simulink model "fec_ber_hw_V2"  (R2020b)
settings: Solver=FixedStepDiscrete  StartTime=0.0  StopTime=T  RelTol=1e-3
values from neighbouring files (symbols this model uses):
  aximm_awgn_reset = 0    [setup.m]
  aximm_bit_count_reset = 0    [setup.m]
  aximm_bits = n_blocks * k    (= 80)    [setup.m]
  aximm_ctrl_word_dec = 0    [setup.m]
  aximm_ctrl_word_enc = 0    [setup.m]
  aximm_enable = 1    [setup.m]
  aximm_length = k * n_blocks    (= 80)    [setup.m]
  aximm_length_dec = n    (= 160)    [setup.m]
  aximm_length_enc = k    (= 80)    [setup.m]
  aximm_llr_mag_reset = 0    [setup.m]
  aximm_llr_scale = (1/noise_var) * llr_scale    (= 1000)    [setup.m]
  aximm_load_dec = 1    [setup.m]
  aximm_load_enc = 1    [setup.m]
  aximm_noise_std = sqrt(noise_var)    [setup.m]
  aximm_reset = 0    [setup.m]
  d = sqrt(-2*log([0:1/4095:1]))    [setup.m]
  fs = 160e6    (= 160000000)    [setup.m]
  generator_polynomial = '''z^13 + z^12 + z^11 + z^8 + 1'''    [setup.m]
  llr_scale = 7.75/7.75    (= 1)    [setup.m]
libraries: simulink x931, hdlsllib x419, commseqgen3 x52, dspsigops x22, commblkcod2 x3, lib_rfsoc_fec x2
(part 1 of 47)
settings Model: Creator=ckb13136  LastModifiedBy=LDM
settings OptimizationCC: BlockReduction=off  ConditionallyExecuteInputs=off  DefaultParameterBehavior=Inlined
settings DebuggingCC: AlgebraicLoopMsg=error  SingleTaskRateTransMsg=error
settings HardwareCC: ProdBitPerPointer=32  ProdBitPerSizeT=32  ProdBitPerPtrDiffT=32  ProdLargestAtomicFloat=None  ProdIntDivRoundTo=Undefined  ProdEndianess=Unspecified  ProdWordSize=32  ProdHWDeviceType=ASIC/FPGA->ASIC/FPGA  TargetBitPerPointer=64  TargetBitPerSizeT=64  TargetBitPerPtrDiffT=64  TargetLongLongMode=on  TargetIntDivRoundTo=Zero  TargetEndianess=LittleEndian  TargetWordSize=64  TargetHWDeviceType=Custom Processor->MATLAB Host Computer  ProdEqTarget=off

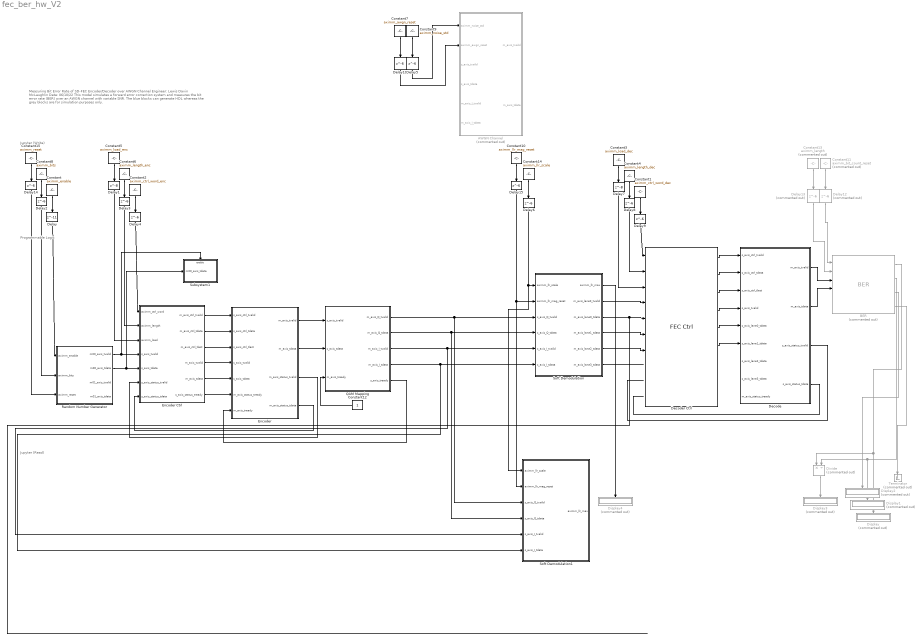
== system fec_ber_hw_V2 ==
  note: Measuring Bit Error Rate of SD-FEC Encoder/Decoder over AWGN Channel
      | Engineer: Lewis Davin McLaughlin
      | Date: 06/10/22
      |
      | This model simulates a forward error correction system and measures the bit error rate (BER) over an AWGN channel with variable SNR. The blue blocks can generate HDL whereas the grey blocks are for simulation purposes only.
  note: Jupyter (Write)
  note: Programmable Logic
  note: Jupyter (Read)
  AWGN Channel : Subsystem  Commented=on  AncestorBlock=lib_rfsoc_fec/AWGN Channel  TreatAsAtomicUnit=on
  BER : lib_rfsoc_fec/BER  Commented=on  SystemSampleTime=-1  VariantActivationTime=update diagram  Latency=0  AutoFrameSizeCalculation=off
  Constant : Constant  Value=aximm_enable  OutDataTypeStr=uint32  SampleTime=1/fs
  Constant1 : Constant  Value=aximm_ctrl_word_dec  OutDataTypeStr=uint32  SampleTime=1/fs
  Constant10 : Constant  Value=aximm_llr_mag_reset  OutDataTypeStr=uint32  SampleTime=1/(fs)
  Constant11 : Constant  Commented=on  Value=aximm_bit_count_reset  OutDataTypeStr=uint32  SampleTime=1/(fs*16)
  Constant12 : Constant  OutDataTypeStr=boolean  SampleTime=1/(fs)
  Constant13 : Constant  Commented=on  Value=aximm_length  OutDataTypeStr=uint32  SampleTime=1/(fs*16)
  Constant14 : Constant  Value=aximm_llr_scale  OutDataTypeStr=fixdt(0,32,22)  SampleTime=1/(fs)
  Constant15 : Constant  Value=aximm_reset  OutDataTypeStr=uint32  SampleTime=1/fs
  Constant2 : Constant  Value=aximm_ctrl_word_enc  OutDataTypeStr=uint32  SampleTime=1/fs
  Constant3 : Constant  Value=aximm_load_dec  OutDataTypeStr=uint32  SampleTime=1/fs
  Constant4 : Constant  Value=aximm_length_dec  OutDataTypeStr=uint32  SampleTime=1/fs
  Constant5 : Constant  Value=aximm_load_enc  OutDataTypeStr=uint32  SampleTime=1/fs
  Constant6 : Constant  Value=aximm_length_enc  OutDataTypeStr=uint32  SampleTime=1/fs
  Constant7 : Constant  Value=aximm_awgn_reset  OutDataTypeStr=uint32  SampleTime=1/(fs*2)
  Constant8 : Constant  Value=aximm_bits  OutDataTypeStr=uint32  SampleTime=1/fs
  Constant9 : Constant  Value=aximm_noise_std  OutDataTypeStr=fixdt(0,32,30)  SampleTime=1/(fs*2)
  Decode : Subsystem
  Decoder Ctrl : lib_rfsoc_fec/FEC Ctrl  SystemSampleTime=-1  VariantActivationTime=update diagram  Latency=0  AutoFrameSizeCalculation=off
  Delay : Delay  DelayLength=11
  Delay1 : Delay  DelayLength=8
  Delay{2..6,8..10,14..15} (10 alike) : Delay  DelayLength=6
  Delay12 : Delay  Commented=on  DelayLength=6
  Delay13 : Delay  Commented=on  DelayLength=6
  Delay7 : Delay  DelayLength=8
  Display{,1..4} (5 alike) : Display  Commented=on
  Divide : Product  Commented=on  Inputs=*/
  Encoder : Subsystem
  Encoder Ctrl : Subsystem  AncestorBlock=lib_rfsoc_fec/FEC Ctrl  TreatAsAtomicUnit=on
  QAM Mapping : Subsystem  AncestorBlock=lib_rfsoc_fec/QAM Mapping  TreatAsAtomicUnit=on
  Random Number Generator : Subsystem  AncestorBlock=lib_rfsoc_fec/Random Number Generator  TreatAsAtomicUnit=on
  Soft Demodulation : Subsystem  AncestorBlock=lib_rfsoc_fec/Soft Demodulation  TreatAsAtomicUnit=on
  Soft Demodulation1 : Subsystem  AncestorBlock=lib_rfsoc_fec/Soft Demodulation  TreatAsAtomicUnit=on
  Subsystem1 : Subsystem
  Terminator : Terminator  Commented=on
  wires:
  BER/3 -> Display2/1
  Soft Demodulation/1(aximm_llr_max) -> Display4/1
  Constant6/1 -> Delay3/1
  Constant7/1 -> Delay10/1
  Encoder Ctrl/2(m_axis_ctrl_tdata) -> Encoder/2(s_axis_ctrl_tdata)
  Constant12/1 -> QAM Mapping/3(m_axis_tready)
  Constant/1 -> Delay/1
  Delay15/1 -> Soft Demodulation1/2(aximm_llr_mag_reset), Soft Demodulation/2(aximm_llr_mag_reset)
  Constant10/1 -> Delay15/1
  Delay10/1 -> AWGN Channel/2(aximm_awgn_reset)
  Delay/1 -> Random Number Generator/1(aximm_enable)
  Delay3/1 -> Encoder Ctrl/2(aximm_length)
  Delay2/1 -> Random Number Generator/2(aximm_bits)
  BER/1 -> Divide/1, Display/1
  Soft Demodulation/2(m_axis_lane0_tvalid) -> Decoder Ctrl/4
  Delay12/1 -> BER/1
  Constant11/1 -> Delay12/1
  BER/2 -> Divide/2, Display1/1
  Encoder Ctrl/5(m_axis_tdata) -> Encoder/5(s_axis_tdata)
  Decoder Ctrl/4 -> Decode/4(s_axis_tvalid)
  Constant2/1 -> Delay4/1
  Constant9/1 -> Delay5/1
  Decode/1(m_axis_tvalid) -> BER/3
  Delay1/1 -> Encoder Ctrl/3(aximm_load)
  Delay4/1 -> Encoder Ctrl/1(aximm_ctrl_word)
  Decode/2(m_axis_tdata) -> BER/4
  Decoder Ctrl/2 -> Decode/2(s_axis_ctrl_tdata)
  Encoder Ctrl/3(m_axis_ctrl_tlast) -> Encoder/3(s_axis_ctrl_tlast)
  Decoder Ctrl/3 -> Decode/3(s_axis_ctrl_tlast)
  Divide/1 -> Display3/1
  Encoder/1(m_axis_tvalid) -> QAM Mapping/1(s_axis_tvalid)
  Delay6/1 -> Soft Demodulation1/1(aximm_llr_scale), Soft Demodulation/1(aximm_llr_scale)
  Encoder Ctrl/4(m_axis_tvalid) -> Encoder/4(s_axis_tvalid)
  Delay5/1 -> AWGN Channel/1(aximm_noise_std)
  Encoder/2(m_axis_tdata) -> QAM Mapping/2(s_axis_tdata)
  Decoder Ctrl/1 -> Decode/1(s_axis_ctrl_tvalid)
  Constant14/1 -> Delay6/1
  Decoder Ctrl/5 -> Decode/5(s_axis_lane0_tdata)
  Constant8/1 -> Delay2/1
  Encoder Ctrl/1(m_axis_ctrl_tvalid) -> Encoder/1(s_axis_ctrl_tvalid)
  Constant5/1 -> Delay1/1
  BER/4 -> Terminator/1
  Constant13/1 -> Delay13/1
  Delay13/1 -> BER/2
  Delay14/1 -> Random Number Generator/3(aximm_reset)
  Constant15/1 -> Delay14/1
  QAM Mapping/5(s_axis_tready) -> Encoder/7(m_axis_tready)
  Random Number Generator/2(m00_axis_tdata) -> Subsystem1/1(m00_axis_tdata), Encoder Ctrl/5(s_axis_tdata)
  Random Number Generator/1(m00_axis_tvalid) -> Subsystem1/Enable, Encoder Ctrl/4(s_axis_tvalid)
  Encoder Ctrl/6(s_axis_status_tready) -> Encoder/6(m_axis_status_tready)
  QAM Mapping/1(m_axis_Q_tvalid) -> Soft Demodulation1/3(s_axis_Q_tvalid), Soft Demodulation/3(s_axis_Q_tvalid)
  QAM Mapping/2(m_axis_Q_tdata) -> Soft Demodulation1/4(s_axis_Q_tdata), Soft Demodulation/4(s_axis_Q_tdata)
  QAM Mapping/3(m_axis_I_tvalid) -> Soft Demodulation1/5(s_axis_I_tvalid), Soft Demodulation/5(s_axis_I_tvalid)
  QAM Mapping/4(m_axis_I_tdata) -> Soft Demodulation1/6(s_axis_I_tdata), Soft Demodulation/6(s_axis_I_tdata)
  Encoder/3(m_axis_status_tvalid) -> Encoder Ctrl/6(s_axis_status_tvalid)
  Encoder/4(m_axis_status_tdata) -> Encoder Ctrl/7(s_axis_status_tdata)
  Soft Demodulation/4(m_axis_lane1_tdata) -> Decoder Ctrl/6
  Soft Demodulation/5(m_axis_lane2_tdata) -> Decoder Ctrl/7
  Soft Demodulation/6(m_axis_lane3_tdata) -> ?
  Delay9/1 -> Decoder Ctrl/1
  Constant4/1 -> Delay8/1
  Constant1/1 -> Delay9/1
  Constant3/1 -> Delay7/1
  Delay8/1 -> Decoder Ctrl/2
  Delay7/1 -> Decoder Ctrl/3
  Decoder Ctrl/6 -> Decode/6(s_axis_lane1_tdata)
  ? -> Decode/7(s_axis_lane2_tdata)
  ? -> Decode/8(s_axis_lane3_tdata)
  Decode/3(s_axis_status_tvalid) -> ?
  Decode/4(s_axis_status_tdata) -> ?
  Soft Demodulation/3(m_axis_lane0_tdata) -> Decoder Ctrl/5

== system fec_ber_hw_V2/AWGN Channel ==
  aximm_noise_std : Inport
  aximm_awgn_reset : Inport  Port=2
  s_axis_tvalid : Inport  Port=3
  s_axis_tdata : Inport  Port=4
  m_axis_I_tvalid : Inport  Port=5
  m_axis_I_tdata : Inport  Port=6
  AWGN Generator : Subsystem
  Add : Sum  OutDataTypeStr=fixdt(1,16,11)  SaturateOnIntegerOverflow=on
  Bit Concat : hdlsllib/Logic and Bit Operations/Bit Concat  numInputs=2
  Bit Slice : hdlsllib/Logic and Bit Operations/Bit Slice  lidx=3  ridx=0
      settings: SourceProductBaseCode=SL
  Bit Slice1 : hdlsllib/Logic and Bit Operations/Bit Slice  lidx=7  ridx=4
      settings: SourceProductBaseCode=SL
  Cast To Boolean : DataTypeConversion  OutDataTypeStr=boolean
  Complex to Real-Imag : ComplexToRealImag
  Data Type Conversion : DataTypeConversion  OutDataTypeStr=fixdt(1,4,0)  ConvertRealWorld=Stored Integer (SI)
  Data Type Conversion1 : DataTypeConversion  OutDataTypeStr=fixdt(1,4,0)  ConvertRealWorld=Stored Integer (SI)
  Delay{,1..5} (6 alike) : Delay
  Downsample{,1..3} (4 alike) : DownSample  N=4  RateOptions=Allow multirate processing
  Real-Imag to Complex : RealImagToComplex
  Repeat : dspsigops/Repeat  N=4  InputProcessing=Columns as channels (frame based)  RateOptions=Allow multirate processing  ic=0  mode=Unused parameter value
      settings: SourceProductName=DSP System Toolbox
  Repeat1 : dspsigops/Repeat  N=4  InputProcessing=Columns as channels (frame based)  RateOptions=Allow multirate processing  ic=0  mode=Unused parameter value
      settings: SourceProductName=DSP System Toolbox
  sample_and_hold : Subsystem
  m_axis_tvalid : Outport
  m_axis_tdata : Outport  Port=2
  wires:
  Cast To Boolean/1 -> Downsample3/1
  aximm_awgn_reset/1 -> Cast To Boolean/1
  Downsample3/1 -> Delay5/1
  Complex to Real-Imag/2 -> Bit Concat/2
  Complex to Real-Imag/1 -> Bit Concat/1
  Bit Concat/1 -> Delay4/1
  Add/1 -> Complex to Real-Imag/1
  Real-Imag to Complex/1 -> Add/1
  Data Type Conversion1/1 -> Real-Imag to Complex/2
  Data Type Conversion/1 -> Real-Imag to Complex/1
  Bit Slice/1 -> Data Type Conversion1/1
  Bit Slice1/1 -> Data Type Conversion/1
  Delay4/1 -> Repeat1/1
  Delay3/1 -> Repeat/1
  Repeat/1 -> m_axis_tvalid/1
  Repeat1/1 -> m_axis_tdata/1
  Delay1/1 -> Bit Slice/1, Bit Slice1/1
  s_axis_tdata/1 -> sample_and_hold/2(data_in)
  s_axis_tvalid/1 -> sample_and_hold/1(valid_in)
  sample_and_hold/2(" data_out") -> Downsample/1
  Delay/1 -> Delay3/1
  Downsample/1 -> Delay1/1
  Downsample1/1 -> Delay/1
  sample_and_hold/1(" valid_out") -> Downsample1/1
  Delay5/1 -> AWGN Generator/2(reset)
  Downsample2/1 -> Delay2/1
  Delay2/1 -> AWGN Generator/1(noise_std)
  aximm_noise_std/1 -> Downsample2/1
  AWGN Generator/1(awgn) -> Add/2

== system fec_ber_hw_V2/Decode ==
  s_axis_ctrl_tvalid : Inport
  s_axis_ctrl_tdata : Inport  Port=2
  s_axis_ctrl_tlast : Inport  Port=3
  s_axis_tvalid : Inport  Port=4
  s_axis_lane0_tdata : Inport  Port=5
  s_axis_lane1_tdata : Inport  Port=6
  s_axis_lane2_tdata : Inport  Port=7
  s_axis_lane3_tdata : Inport  Port=8
  m_axis_status_tready : Inport  Port=9
  Bit Slice{,2,4,6} (4 alike) : hdlsllib/Logic and Bit Operations/Bit Slice  lidx=63  ridx=0
      settings: SourceProductBaseCode=SL
  Bit Slice{1,3,5,7} (4 alike) : hdlsllib/Logic and Bit Operations/Bit Slice  lidx=127  ridx=64
      settings: SourceProductBaseCode=SL
  Cast To Boolean : DataTypeConversion  OutDataTypeStr=boolean
  Constant1 : Constant  Value=aximm_bits  OutDataTypeStr=uint32  SampleTime=1/fs
  Constant3 : Constant  Value=0  OutDataTypeStr=uint32  SampleTime=1/(16*fs)
  Constant4 : Constant  Value=0  OutDataTypeStr=boolean  SampleTime=1/(16*fs)
  Constant8 : Constant  Value=aximm_bits  OutDataTypeStr=uint32  SampleTime=1/fs
  Data Type Conversion : DataTypeConversion  OutDataTypeStr=fixdt(1,6,2)  ConvertRealWorld=Stored Integer (SI)
  Gain : Gain  Gain=1/llr_scale
  MATLAB Function3 : MATLAB Function  TreatAsAtomicUnit=on
  MATLAB Function5 : MATLAB Function  TreatAsAtomicUnit=on
  NOT2 : Logic  Operator=NOT  IconShape=distinctive  AllPortsSameDT=off  OutDataTypeStr=boolean
  Subsystem : Subsystem
  Subsystem1 : Subsystem
  Terminator{,1..3} (4 alike) : Terminator
  m_axis_tvalid : Outport
  m_axis_tdata : Outport  Port=2
  s_axis_status_tvalid : Outport  Port=3
  s_axis_status_tdata : Outport  Port=4
  wires:
  Data Type Conversion/1 -> Gain/1
  ? -> Data Type Conversion/1
  Gain/1 -> ?
  s_axis_ctrl_tvalid/1 -> Terminator/1
  s_axis_ctrl_tdata/1 -> Terminator1/1
  s_axis_ctrl_tlast/1 -> Terminator2/1
  m_axis_status_tready/1 -> Terminator3/1
  Constant4/1 -> s_axis_status_tvalid/1
  Constant3/1 -> s_axis_status_tdata/1
  NOT2/1 -> MATLAB Function5/3(frame)
  Subsystem/1(Out1) -> NOT2/1
  s_axis_tvalid/1 -> MATLAB Function3/2(valid)
  Constant8/1 -> MATLAB Function3/1(bits)
  MATLAB Function3/2(frame_out) -> Subsystem/1(In1)
  MATLAB Function3/1(valid_out) -> Cast To Boolean/1
  Bit Slice/1 -> MATLAB Function3/3(lane_0)
  Bit Slice1/1 -> MATLAB Function3/4(lane_1)
  s_axis_lane0_tdata/1 -> Bit Slice1/1, Bit Slice/1
  s_axis_lane1_tdata/1 -> Bit Slice2/1, Bit Slice3/1
  Bit Slice3/1 -> MATLAB Function3/6(lane_3)
  Bit Slice2/1 -> MATLAB Function3/5(lane_2)
  s_axis_lane2_tdata/1 -> Bit Slice5/1, Bit Slice4/1
  Bit Slice4/1 -> MATLAB Function3/7(lane_4)
  Bit Slice5/1 -> MATLAB Function3/8(lane_5)
  Bit Slice7/1 -> MATLAB Function3/10(lane_7)
  Bit Slice6/1 -> MATLAB Function3/9(lane_6)
  s_axis_lane3_tdata/1 -> Bit Slice7/1, Bit Slice6/1
  Constant1/1 -> MATLAB Function5/1(bits)
  MATLAB Function5/1(tvalid) -> Subsystem1/Enable
  MATLAB Function5/2(lane_0) -> Subsystem1/1(lane_0)
  Cast To Boolean/1 -> MATLAB Function5/2(valid), Subsystem/Enable

== system fec_ber_hw_V2/Encoder ==
  s_axis_ctrl_tvalid : Inport
  s_axis_ctrl_tdata : Inport  Port=2
  s_axis_ctrl_tlast : Inport  Port=3
  s_axis_tvalid : Inport  Port=4
  s_axis_tdata : Inport  Port=5
  m_axis_status_tready : Inport  Port=6
  m_axis_tready : Inport  Port=7
  Cast To Double : DataTypeConversion  OutDataTypeStr=double
  Constant1 : Constant  Value=aximm_bits * 2  OutDataTypeStr=uint32  SampleTime=1/(fs)
  Constant2 : Constant  Value=0  OutDataTypeStr=boolean  SampleTime=1/fs
  Constant3 : Constant  Commented=on  Value=aximm_bits  OutDataTypeStr=uint32  SampleTime=1/fs
  Constant4 : Constant  Value=0  OutDataTypeStr=boolean  SampleTime=1/fs
  Constant8 : Constant  Value=aximm_bits  OutDataTypeStr=uint32  SampleTime=1/(fs)
  Encode : Subsystem
  MATLAB Function : MATLAB Function  Commented=on  TreatAsAtomicUnit=on
  MATLAB Function3 : MATLAB Function  TreatAsAtomicUnit=on
  MATLAB Function4 : MATLAB Function  TreatAsAtomicUnit=on
  MATLAB Function5 : MATLAB Function  Commented=on  TreatAsAtomicUnit=on
  NOT2 : Logic  Commented=on  Operator=NOT  IconShape=distinctive  AllPortsSameDT=off  OutDataTypeStr=boolean
  Subsystem : Subsystem  Commented=on
  Subsystem1 : Subsystem  Commented=on
  Terminator{,1..4} (5 alike) : Terminator
  m_axis_tvalid : Outport
  m_axis_tdata : Outport  Port=2
  m_axis_status_tvalid : Outport  Port=3
  m_axis_status_tdata : Outport  Port=4
  wires:
  Constant4/1 -> m_axis_status_tvalid/1
  s_axis_ctrl_tvalid/1 -> Terminator/1
  s_axis_ctrl_tdata/1 -> Terminator1/1
  s_axis_ctrl_tlast/1 -> Terminator2/1
  m_axis_status_tready/1 -> Terminator3/1
  m_axis_tready/1 -> Terminator4/1
  MATLAB Function3/2(frame_out) -> Encode/1(frame_out)
  s_axis_tvalid/1 -> MATLAB Function3/2(valid)
  s_axis_tdata/1 -> MATLAB Function3/3(lane_0)
  Constant8/1 -> MATLAB Function3/1(bits)
  Encode/1(frame) -> Cast To Double/1, MATLAB Function4/3(frame)
  MATLAB Function4/1(tvalid) -> m_axis_tvalid/1
  Constant1/1 -> MATLAB Function4/1(bits)
  MATLAB Function4/2(lane_0) -> m_axis_tdata/1
  Constant2/1 -> m_axis_status_tdata/1
  NOT2/1 -> MATLAB Function5/3(frame)
  MATLAB Function5/1(tvalid) -> Subsystem1/Enable
  Constant3/1 -> MATLAB Function5/1(bits)
  Subsystem/1(Out1) -> NOT2/1
  MATLAB Function3/1(valid_out) -> Encode/Enable, Subsystem/Enable, MATLAB Function5/2(valid), MATLAB Function4/2(valid)
  Cast To Double/1 -> MATLAB Function/1(u)
  MATLAB Function5/2(lane_0) -> Subsystem1/1(In1)
  MATLAB Function/1(y) -> Subsystem/1(frame)

== system fec_ber_hw_V2/Encoder Ctrl ==
  aximm_ctrl_word : Inport
  aximm_length : Inport  Port=2
  aximm_load : Inport  Port=3
  s_axis_tvalid : Inport  Port=4
  s_axis_tdata : Inport  Port=5
  s_axis_status_tvalid : Inport  Port=6
  s_axis_status_tdata : Inport  Port=7
  Chart : Stateflow chart  TreatAsAtomicUnit=on
      settings: PortSchema="{\"entries\":[{\"content\":{\"sides\":[{\"content\":{\"connectorIds\":[\"In1\",\"In2\",\"In3\",\"In4\",\"In5\"]},\"type\":\"ConnectorPlacement.EquallySpacedRectSide\",\"uuid\":\"96b1e0a6-9243-45af-ad4c-9b6bdb766973\"},{\"content\":{\"connectorIds\":[\"Out1\",\"Out2\",\"Out3\",\"Out4\",\"Out7\",\"Out5\",\"Out6\"],\"side\":\"RIGHT\"},\"type\":\"ConnectorPlacement.EquallySpacedRectSide\",\"uuid\":\"a962d190-29ee-4ef5-b85e-0d462d6476b7\"},{\"content\":{\"connectorIds\":[],\"side\":\"TOP\"},\"type\":\"ConnectorPlacement.EquallySpacedRectSide\",\"uuid\":\"6028541f-0eff-4bfb-a496-920287fbe05d\"},{\"content\":{\"connectorIds\":[],\"side\":\"HIDDEN\"},\"type\":\"ConnectorPlacement.EquallySpacedRectSide\",\"uuid\":\"2bd272f9-f96d-47a2-bf8a-d251a31e3228\"}]},\"type\":\"ConnectorPlacement.EquallySpacedConnector\",\"uuid\":\"9912cff3-58c1-4038-915e-716fff51edba\"}],\"packageUris\":[\"http://schema.mathworks.com/mf0/Connector/R2020b\"],\"version\":\"1.0\"}"
  Delay : Delay  DelayLength=1
  Delay1 : Delay  DelayLength=1
  Rising Edge : Subsystem
  Terminator : Terminator
  Terminator1 : Terminator
  Terminator2 : Terminator
  m_axis_ctrl_tvalid : Outport
  m_axis_ctrl_tdata : Outport  Port=2
  m_axis_ctrl_tlast : Outport  Port=3
  m_axis_tvalid : Outport  Port=4
  m_axis_tdata : Outport  Port=5
  s_axis_status_tready : Outport  Port=6
  wires:
  Rising Edge/1(Out1) -> Chart/3(load)
  aximm_load/1 -> Rising Edge/1(In1)
  Delay1/1 -> m_axis_tdata/1
  Chart/7(m_axis_tdata) -> Delay1/1
  s_axis_status_tdata/1 -> Terminator2/1
  s_axis_status_tvalid/1 -> Terminator1/1
  Delay/1 -> m_axis_tvalid/1
  Chart/1(m_axis_ctrl_tvalid) -> m_axis_ctrl_tvalid/1
  Chart/5(s_axis_status_tready) -> s_axis_status_tready/1
  Chart/4(m_axis_tvalid) -> Delay/1
  Chart/2(m_axis_ctrl_tdata) -> m_axis_ctrl_tdata/1
  aximm_ctrl_word/1 -> Chart/1(ctrl_word)
  s_axis_tdata/1 -> Chart/5(s_axis_tdata)
  s_axis_tvalid/1 -> Chart/4(s_axis_tvalid)
  aximm_length/1 -> Chart/2(block_length)
  Chart/6(state) -> Terminator/1
  Chart/3(m_axis_ctrl_tlast) -> m_axis_ctrl_tlast/1

== system fec_ber_hw_V2/QAM Mapping ==
  s_axis_tvalid : Inport
  s_axis_tdata : Inport  Port=2
  m_axis_tready : Inport  Port=3
  Buffer : Subsystem
  QAM Mapping : Subsystem
  Terminator : Terminator
  m_axis_Q_tvalid : Outport
  m_axis_Q_tdata : Outport  Port=2
  m_axis_I_tvalid : Outport  Port=3
  m_axis_I_tdata : Outport  Port=4
  s_axis_tready : Outport  Port=5
  wires:
  Buffer/3(s_axis_tready) -> s_axis_tready/1
  s_axis_tvalid/1 -> Buffer/1(s_axis_tvalid)
  s_axis_tdata/1 -> Buffer/2(s_axis_tdata)
  m_axis_tready/1 -> Terminator/1
  QAM Mapping/1(Q symbols) -> m_axis_Q_tdata/1
  Buffer/1(" m_axis_tvalid") -> QAM Mapping/Enable, m_axis_I_tvalid/1, m_axis_Q_tvalid/1
  Buffer/2(" m_axis_tdata") -> QAM Mapping/1(bits lane0)
  QAM Mapping/2(I symbols) -> m_axis_I_tdata/1

== system fec_ber_hw_V2/Random Number Generator ==
  aximm_enable : Inport
  aximm_bits : Inport  Port=2
  aximm_reset : Inport  Port=3
  Cast To Boolean1 : DataTypeConversion  OutDataTypeStr=boolean
  Delay1 : Delay  DelayLength=1
  Random Number Generator : Subsystem  mask{bits=32, gen_poly=generator_polynomial}
      mask prompts: bits "Data Bits:"; gen_poly "Generator Polynomial:"
      mask init:
      | random_gen = gcb;
      | 
      | %set_param(random_gen, 'LinkStatus', 'none');
      | 
      | block_handles = Simulink.findBlocks(gcb);
      | block_names = getfullname(block_handles);
      | 
      | out_block = sprintf('%s/data', random_gen);
      | in_block = sprintf('%s/reset', random_gen);
      | enable_block = sprintf('%s/enable', random_gen);
      | 
      | keep_blocks = {out_block, in_block, enable_block};
      | 
      | for i = 1:length(block_names)
      |     if ~ismember(block_names{i}, keep_blocks)
      |         delete_block(block_names{i});
      |     end
      | end
      | delete_line(find_system(random_gen,'LookUnderMasks', 'all','FindAll','on','type','line'));
      | 
      | % Add all PN Sequence Generators 
      | for bit = 1:bits
      |     current_block = sprintf('%s/bit%d', random_gen, bit-1);
      |     add_block('commseqgen3/PN Sequence Generator', current_block);
      |     position = get_param(current_block, 'position');
      |     if bit == 1
      |         start_position = position;
      |     end
      |     new_position = position + ([0 60 0 60] * (bit-1));
      |     set_param(current_block, 'position', new_position);
      |     set_param(current_block, 'outDataType', 'boolean');
      |     set_param(current_block, 'reset', 'on');
      |     set_param(current_block, 'Ts', '-1');
      |     set_param(current_block, 'poly', gen_poly);
      |     
      |     val = dec2bin(randi(2^13 - 1), 13);
      |     str = '[';
      |     for i = 1:13
      |         str(end+1:end+2) = [' ' (val(i))];
      |     end
      |     str(end+1) = ']';
      |     set_param(current_block, 'ini_sta', str);
      | end
      | 
      | % Add the Bit Concat
      | concat_block = sprintf('%s/concat', random_gen);
      | add_block('hdlsllib/Logic and Bit Operations/Bit Concat', concat_block);
      | set_param(concat_block, 'numInputs', num2str(bits));
      | position = new_position + [150 0 150 0];
      | position(2) = start_position(2);
      | set_param(concat_block, 'position', position);
      | 
      | % Add Input and Outputs
      | out_position = get_param(out_block, 'position');
      | height = out_position(4) - out_position(2);
      | width = out_position(3) - out_position(1);
      | middle_h = (position(4) - position(2))/2 + position(2);
      | out_position = [position(1) + 150, middle_h - height/2, position(1) + 150 + width, middle_h + height/2];
      | set_param(out_block, 'position', out_position);
      | 
      | in_position = [position(1) - 300, middle_h - height/2, position(1) - 300 + width, middle_h + height/2];
      | set_param(in_block, 'position', in_position);
      | 
      | enable_position = get_param(enable_block, 'position');
      | set_param(enable_block, 'position', enable_position - [0 100 0 100]);
      | 
      | % Connect Ports
      | for bit = 1:bits
      |     add_line(random_gen,'reset/1', sprintf('bit%d/1', bit-1));
      |     add_line(random_gen,sprintf('bit%d/1', bit-1), sprintf('concat/%d', bit));
      | end
      | add_line(random_gen,'concat/1','data/1');
      mask DialogControl DescGroupVar Prompt: N-Bit Random Number Generator
      mask DialogControl DescTextVar Prompt: This block will create a n-bit random number generator. Provide a polynomial and the number of bits. Information on polynomials for maximal LFSRs can be found:  https://en.wikipedia.org/wiki/Linear-feedback_shift_register For example: ''z^13 + z^12 + z^11 + z^8 + 1''
  concat : Subsystem
  rising_edge : Subsystem
  tvalid hold : Subsystem
  m00_axis_tvalid : Outport
  m00_axis_tdata : Outport  Port=2
  m01_axis_tvalid : Outport  Port=3
  m01_axis_tdata : Outport  Port=4
  wires:
  concat/1(d_out) -> m01_axis_tdata/1, m00_axis_tdata/1
  aximm_reset/1 -> Cast To Boolean1/1
  aximm_enable/1 -> rising_edge/1(in)
  rising_edge/1(pulse) -> tvalid hold/1(trigger)
  aximm_bits/1 -> tvalid hold/2(comparator)
  Cast To Boolean1/1 -> Random Number Generator/1(reset)
  tvalid hold/1(enable) -> Delay1/1, Random Number Generator/Enable, concat/1(en)
  tvalid hold/2(diff) -> concat/2(diff)
  Random Number Generator/1(data) -> concat/3(d_in)
  Delay1/1 -> m01_axis_tvalid/1, m00_axis_tvalid/1

== system fec_ber_hw_V2/Soft Demodulation ==
  aximm_llr_scale : Inport
  aximm_llr_mag_reset : Inport  Port=2
  s_axis_Q_tvalid : Inport  Port=3
  s_axis_Q_tdata : Inport  Port=4
  s_axis_I_tvalid : Inport  Port=5
  s_axis_I_tdata : Inport  Port=6
  Bit Concat : hdlsllib/Logic and Bit Operations/Bit Concat  numInputs=2
  Bit Slice : hdlsllib/Logic and Bit Operations/Bit Slice  lidx=23  ridx=0
      settings: SourceProductBaseCode=SL
  Bit Slice1 : hdlsllib/Logic and Bit Operations/Bit Slice  lidx=71  ridx=48
      settings: SourceProductBaseCode=SL
  Bit Slice2 : hdlsllib/Logic and Bit Operations/Bit Slice  lidx=47  ridx=0
      settings: SourceProductBaseCode=SL
  Bit Slice3 : hdlsllib/Logic and Bit Operations/Bit Slice  lidx=95  ridx=48
      settings: SourceProductBaseCode=SL
  Bit Slice4 : hdlsllib/Logic and Bit Operations/Bit Slice  lidx=47  ridx=0
      settings: SourceProductBaseCode=SL
  Bit Slice5 : hdlsllib/Logic and Bit Operations/Bit Slice  lidx=95  ridx=48
      settings: SourceProductBaseCode=SL
  Bit Slice6 : hdlsllib/Logic and Bit Operations/Bit Slice  lidx=47  ridx=0
      settings: SourceProductBaseCode=SL
  Bit Slice7 : hdlsllib/Logic and Bit Operations/Bit Slice  lidx=95  ridx=48
      settings: SourceProductBaseCode=SL
  Bit Slice8 : hdlsllib/Logic and Bit Operations/Bit Slice  lidx=23  ridx=0
      settings: SourceProductBaseCode=SL
  Cast To Boolean : DataTypeConversion  Commented=on  OutDataTypeStr=boolean
  MATLAB Function : MATLAB Function  Commented=on  TreatAsAtomicUnit=on
  SSR Soft Demodulation Lane 0 : Subsystem  mask{ssr=8}
      mask init:
      | top_block = gcb;
      | 
      | block_names = find_system(top_block, 'LookUnderMasks','on', 'SearchDepth','1');
      | 
      | in_valid = sprintf('%s/valid', top_block);
      | in_real = sprintf('%s/real', top_block);
      | in_imag = sprintf('%s/imag', top_block);
      | in_scale = sprintf('%s/scale', top_block);
      | out_llr = sprintf('%s/llr', top_block);
      | soft_demod_block = sprintf('%s/Soft Demodulation 0', top_block);
      | 
      | keep_blocks = {top_block,in_valid,in_real,in_imag,in_scale,soft_demod_block,out_llr};
      | 
      | for i = 1:length(block_names)
      |     if ~ismember(block_names{i}, keep_blocks)
      |         delete_block(block_names{i});
      |     end
      | end
      | delete_line(find_system(top_block,'LookUnderMasks', 'all','SearchDepth', '1', 'FindAll','on','type','line'));
      | 
      | % Add Soft Demodulation Blocks
      | pos = get_param(soft_demod_block, 'position');
      | new_pos = pos;
      | for i = 1:ssr-1
      |     new_block = sprintf('%s%d', soft_demod_block(1:end-1), i);
      |     add_block(soft_demod_block, new_block);
      |     new_pos = pos + ([0 150 0 150] * i);
      |     set_param(new_block, 'position', new_pos);
      |     set_param(new_block, 'n', num2str(ssr-i));
      | end
      | 
      | % Add the Bit Concat
      | concat_block = sprintf('%s/concat', top_block);
      | add_block('hdlsllib/Logic and Bit Operations/Bit Concat', concat_block);
      | set_param(concat_block, 'numInputs', num2str(ssr));
      | concat_position = new_pos + [275 0 175 0];
      | concat_position(2) = pos(2);
      | set_param(concat_block, 'position', concat_position);
      | 
      | % Reposition Output
      | out_position = get_param(out_llr, 'position');
      | height = out_position(4) - out_position(2);
      | width = out_position(3) - out_position(1);
      | middle_h = (concat_position(4) - concat_position(2))/2 + concat_position(2);
      | out_position = [concat_position(1) + 175, middle_h - height/2, concat_position(1) + 175 + width, middle_h + height/2];
      | set_param(out_llr, 'position', out_position);
      | 
      | % Connect Ports
      | for i = 1:ssr
      |     add_line(top_block,'valid/1',sprintf('Soft Demodulation %d/1',i-1));
      |     add_line(top_block,'real/1',sprintf('Soft Demodulation %d/2',i-1));
      |     add_line(top_block,'imag/1',sprintf('Soft Demodulation %d/3',i-1));
      |     add_line(top_block,'scale/1',sprintf('Soft Demodulation %d/4',i-1));
      |     
      |     add_line(top_block,sprintf('Soft Demodulation %d/1',i-1),sprintf('concat/%d', i));
      | end
      | add_line(top_block,'concat/1','llr/1');
  SSR Soft Demodulation Lane 1 : Subsystem  mask{ssr=16}
      mask init: same as fec_ber_hw_V2/Soft Demodulation/SSR Soft Demodulation Lane 0
  SSR Soft Demodulation Lane 2 : Subsystem  mask{ssr=16}
      mask init: same as fec_ber_hw_V2/Soft Demodulation/SSR Soft Demodulation Lane 0
  SSR Soft Demodulation Lane 3 : Subsystem  mask{ssr=16}
      mask init: same as fec_ber_hw_V2/Soft Demodulation/SSR Soft Demodulation Lane 0
  SSR Soft Demodulation Lane 4 : Subsystem  mask{ssr=8}
      mask init: same as fec_ber_hw_V2/Soft Demodulation/SSR Soft Demodulation Lane 0
  Subsystem : Subsystem
  byte_count : Subsystem  AncestorBlock=lib_rfsoc_fec/Random Number Generator/byte_count
  interface_creator : Subsystem  AncestorBlock=lib_rfsoc_fec/Random Number Generator/interface_creator
  aximm_llr_max : Outport
  m_axis_lane0_tvalid : Outport  Port=2
  m_axis_lane0_tdata : Outport  Port=3
  m_axis_lane1_tdata : Outport  Port=4
  m_axis_lane2_tdata : Outport  Port=5
  m_axis_lane3_tdata : Outport  Port=6
  wires:
  Cast To Boolean/1 -> MATLAB Function/2(reset)
  aximm_llr_mag_reset/1 -> byte_count/1(reset), Cast To Boolean/1
  MATLAB Function/1(y) -> aximm_llr_max/1
  SSR Soft Demodulation Lane 0/1(llr) -> Subsystem/1(In1), m_axis_lane0_tdata/1
  s_axis_I_tvalid/1 -> byte_count/2(en), interface_creator/4(valid)
  byte_count/2(enable) -> interface_creator/3(en)
  byte_count/1(count) -> interface_creator/2(count)
  s_axis_I_tdata/1 -> Bit Concat/2
  s_axis_Q_tdata/1 -> Bit Concat/1
  Bit Concat/1 -> interface_creator/1(data_in)
  interface_creator/4(lane_1_tdata) -> Bit Slice2/1, Bit Slice3/1
  Bit Slice2/1 -> SSR Soft Demodulation Lane 1/2(real)
  Bit Slice3/1 -> SSR Soft Demodulation Lane 1/3(imag)
  interface_creator/3(lane_1_tvalid) -> SSR Soft Demodulation Lane 1/1(valid)
  interface_creator/5(lane_2_tvalid) -> SSR Soft Demodulation Lane 2/1(valid)
  Bit Slice5/1 -> SSR Soft Demodulation Lane 2/3(imag)
  Bit Slice4/1 -> SSR Soft Demodulation Lane 2/2(real)
  interface_creator/6(lane_2_tdata) -> Bit Slice5/1, Bit Slice4/1
  interface_creator/8(lane_3_tdata) -> Bit Slice6/1, Bit Slice7/1
  Bit Slice6/1 -> SSR Soft Demodulation Lane 3/2(real)
  Bit Slice7/1 -> SSR Soft Demodulation Lane 3/3(imag)
  interface_creator/7(lane_3_tvalid) -> SSR Soft Demodulation Lane 3/1(valid)
  aximm_llr_scale/1 -> SSR Soft Demodulation Lane 1/4(scale), SSR Soft Demodulation Lane 3/4(scale), SSR Soft Demodulation Lane 2/4(scale), SSR Soft Demodulation Lane 0/4(scale)
  SSR Soft Demodulation Lane 1/1(llr) -> m_axis_lane1_tdata/1
  SSR Soft Demodulation Lane 2/1(llr) -> m_axis_lane2_tdata/1
  SSR Soft Demodulation Lane 3/1(llr) -> m_axis_lane3_tdata/1
  interface_creator/1(lane_0_tvalid) -> Subsystem/Enable, m_axis_lane0_tvalid/1, SSR Soft Demodulation Lane 0/1(valid)
  Bit Slice/1 -> SSR Soft Demodulation Lane 0/2(real)
  Bit Slice1/1 -> SSR Soft Demodulation Lane 0/3(imag)
  interface_creator/2(lane_0_tdata) -> Bit Slice8/1, Bit Slice/1, Bit Slice1/1
  Bit Slice8/1 -> SSR Soft Demodulation Lane 4/2(real)

== system fec_ber_hw_V2/Soft Demodulation1 ==
  aximm_llr_scale : Inport
  aximm_llr_mag_reset : Inport  Port=2
  s_axis_Q_tvalid : Inport  Port=3
  s_axis_Q_tdata : Inport  Port=4
  s_axis_I_tvalid : Inport  Port=5
  s_axis_I_tdata : Inport  Port=6
  Bit Slice : hdlsllib/Logic and Bit Operations/Bit Slice  lidx=5  ridx=0
      settings: SourceProductBaseCode=SL
  Cast To Boolean : DataTypeConversion  Commented=on  OutDataTypeStr=boolean
  Data Type Conversion : DataTypeConversion  OutDataTypeStr=fixdt(1,6,2)  ConvertRealWorld=Stored Integer (SI)
  MATLAB Function : MATLAB Function  Commented=on  TreatAsAtomicUnit=on
  MATLAB Function1 : MATLAB Function  TreatAsAtomicUnit=on
  MATLAB Function2 : MATLAB Function  TreatAsAtomicUnit=on
  Repeat{,1..3} (4 alike) : dspsigops/Repeat  N=16  InputProcessing=Columns as channels (frame based)  RateOptions=Allow multirate processing  ic=0  mode=Unused parameter value
      settings: SourceProductName=DSP System Toolbox
  Repeat{4..12} (9 alike) : dspsigops/Repeat  N=4  InputProcessing=Columns as channels (frame based)  RateOptions=Allow multirate processing  ic=0  mode=Unused parameter value
      settings: SourceProductName=DSP System Toolbox
  Reshape : Reshape  OutputDimensionality=Row vector (2-D)
  SSR : Subsystem
  Soft Demodulation 0 : Subsystem  mask{w=3, f=0, n=1}
  Soft Demodulation 1 : Subsystem  mask{w=3, f=0, n=1}
  Subsystem : Subsystem
  aximm_llr_max : Outport
  wires:
  s_axis_Q_tdata/1 -> MATLAB Function2/3(data_q), Repeat/1
  s_axis_I_tdata/1 -> SSR/1(data_wide), MATLAB Function2/2(data_i), Repeat1/1
  s_axis_I_tvalid/1 -> Repeat10/1, MATLAB Function2/1(valid), Repeat3/1
  MATLAB Function/1(y) -> aximm_llr_max/1
  aximm_llr_mag_reset/1 -> Cast To Boolean/1
  Cast To Boolean/1 -> MATLAB Function/2(reset)
  Repeat1/1 -> MATLAB Function1/2(data_i)
  Repeat/1 -> MATLAB Function1/3(data_q)
  MATLAB Function1/1(dout_i) -> Repeat4/1
  MATLAB Function1/2(dout_q) -> Repeat5/1
  aximm_llr_scale/1 -> Repeat11/1, Repeat2/1
  Repeat2/1 -> Repeat6/1
  Repeat3/1 -> MATLAB Function1/1(valid), Repeat7/1
  Soft Demodulation 0/1(LLR Values) -> Bit Slice/1
  Repeat4/1 -> Soft Demodulation 0/2(real)
  Repeat5/1 -> Soft Demodulation 0/3(imag)
  Repeat6/1 -> Soft Demodulation 0/4(LLR Scale)
  Repeat7/1 -> Soft Demodulation 0/1(valid), Subsystem/Enable
  Bit Slice/1 -> Data Type Conversion/1
  Data Type Conversion/1 -> Subsystem/1(In1)
  MATLAB Function2/1(frame_i) -> Repeat8/1
  MATLAB Function2/2(frame_q) -> Repeat9/1
  Repeat8/1 -> Soft Demodulation 1/2(real)
  Repeat9/1 -> Soft Demodulation 1/3(imag)
  Repeat10/1 -> Soft Demodulation 1/1(valid)
  Repeat11/1 -> Soft Demodulation 1/4(LLR Scale)
  Soft Demodulation 1/1(LLR Values) -> ?
  SSR/1(data_ssr) -> Reshape/1
  Reshape/1 -> Repeat12/1
  Repeat12/1 -> ?

== system fec_ber_hw_V2/Subsystem1 ==
  m00_axis_tdata : Inport
  Enable : EnablePort
  To Workspace : ToWorkspace  VariableName=num  SampleTime=-1
      settings: Save2DSignal=2-D array (concatenate along first dimension)
  wires:
  m00_axis_tdata/1 -> To Workspace/1

== system fec_ber_hw_V2/AWGN Channel/AWGN Generator ==
  noise_std : Inport
  reset : Inport  Port=2
  1-D Lookup Table : Lookup_n-D  NumberOfTableDimensions=1  BreakpointsForDimension1=[0:4095]  BreakpointsForDimension1DataTypeStr=fixdt(0,12,0)  IndexSearchMethod=Evenly spaced points  Table=d  InterpMethod=Flat  ExtrapMethod=Clip  DiagnosticForOutOfRangeInput=Error  InternalRulePriority=Speed  OutDataTypeStr=fixdt(1,18,14)  RndMeth=Simplest  InputSameDT=on
  Cosine Lookup : Lookup_n-D  NumberOfTableDimensions=1  BreakpointsForDimension1=[0:255]  IndexSearchMethod=Evenly spaced points  Table=cos([0:255]*2*pi/256)  InterpMethod=Flat  ExtrapMethod=Clip  DiagnosticForOutOfRangeInput=Error  UseLastTableValue=on  OutDataTypeStr=fixdt(1,16,14)  RndMeth=Simplest  InputSameDT=on
  Data Type Conversion : DataTypeConversion  OutDataTypeStr=fixdt(0,16,14)  RndMeth=Round  SaturateOnIntegerOverflow=on
  Gain : Gain  Gain=0.7  OutDataTypeStr=fixdt(1,15,11)  RndMeth=Nearest  SaturateOnIntegerOverflow=on
  Product : Product  OutDataTypeStr=fixdt(1,17,14)  RndMeth=Round  SaturateOnIntegerOverflow=on
  Product1 : Product  OutDataTypeStr=fixdt(1,17,14)  RndMeth=Round  SaturateOnIntegerOverflow=on
  Product3 : Product  OutDataTypeStr=fixdt(1,18,14)  RndMeth=Round
  Real-Imag to Complex1 : RealImagToComplex
  Sine Lookup : Lookup_n-D  NumberOfTableDimensions=1  BreakpointsForDimension1=[0:255]  IndexSearchMethod=Evenly spaced points  Table=sin([0:255]*2*pi/256)  InterpMethod=Flat  ExtrapMethod=Clip  DiagnosticForOutOfRangeInput=Error  UseLastTableValue=on  OutDataTypeStr=fixdt(1,16,14)  RndMeth=Simplest  InputSameDT=on
  Subsystem3 : Subsystem
  awgn : Outport
  wires:
  Data Type Conversion/1 -> Product3/1
  Real-Imag to Complex1/1 -> Product3/2
  Gain/1 -> awgn/1
  Cosine Lookup/1 -> Product1/1
  Subsystem3/1(LFSR_G) -> Sine Lookup/1, Cosine Lookup/1
  1-D Lookup Table/1 -> Product/2, Product1/2
  Subsystem3/2(LFSR_F) -> 1-D Lookup Table/1
  reset/1 -> Subsystem3/1(Reset)
  Sine Lookup/1 -> Product/1
  Product3/1 -> Gain/1
  Product/1 -> Real-Imag to Complex1/2
  Product1/1 -> Real-Imag to Complex1/1
  noise_std/1 -> Data Type Conversion/1

== system fec_ber_hw_V2/AWGN Channel/sample_and_hold ==
  valid_in : Inport
  data_in : Inport  Port=2
  Sample and Hold : dspsigops/Sample and Hold  trig=Rising edge  initCond=0  latchinput=off
  tvalid hold : Subsystem
  " valid_out" : Outport
  " data_out" : Outport  Port=2
  wires:
  Sample and Hold/1 -> " data_out"/1
  data_in/1 -> Sample and Hold/1
  tvalid hold/1(" ") -> " valid_out"/1
  valid_in/1 -> Sample and Hold/Trigger, tvalid hold/1(In1)

== system fec_ber_hw_V2/Decode/Subsystem ==
  In1 : Inport
  Enable : EnablePort
  LDPC Decoder : commblkcod2/LDPC Decoder  ParityCheckMat=parity_sparse  OutputFmt=Information part  DecisionType=Hard decision  OutputDataType=boolean  NumIter=64  DoParityCheck=on  OutputNumIter=off  OutputFinalChecks=off
      settings: SourceProductBaseCode=CM
  Out1 : Outport
  wires:
  LDPC Decoder/1 -> Out1/1
  In1/1 -> LDPC Decoder/1

== system fec_ber_hw_V2/Decode/Subsystem1 ==
  lane_0 : Inport
  Enable : EnablePort
  To Workspace : ToWorkspace  VariableName=decoded  SampleTime=-1
      settings: Save2DSignal=2-D array (concatenate along first dimension)
  wires:
  lane_0/1 -> To Workspace/1

== system fec_ber_hw_V2/Encoder/Encode ==
  frame_out : Inport
  Enable : EnablePort
  Cast To Boolean1 : DataTypeConversion  OutDataTypeStr=boolean
  Cast To Double : DataTypeConversion  OutDataTypeStr=double
  LDPC Encoder1 : commblkcod2/LDPC Encoder  ParityCheckMat=parity_sparse
      settings: SourceProductBaseCode=CM
  frame : Outport
  wires:
  LDPC Encoder1/1 -> Cast To Boolean1/1
  Cast To Boolean1/1 -> frame/1
  Cast To Double/1 -> LDPC Encoder1/1
  frame_out/1 -> Cast To Double/1

== system fec_ber_hw_V2/Encoder/Subsystem ==
  frame : Inport
  Enable : EnablePort
  LDPC Decoder : commblkcod2/LDPC Decoder  ParityCheckMat=parity_sparse  OutputFmt=Information part  DecisionType=Hard decision  OutputDataType=boolean  NumIter=64  DoParityCheck=on  OutputNumIter=off  OutputFinalChecks=off
      settings: SourceProductBaseCode=CM
  Out1 : Outport
  wires:
  LDPC Decoder/1 -> Out1/1
  frame/1 -> LDPC Decoder/1

== system fec_ber_hw_V2/Encoder/Subsystem1 ==
  In1 : Inport
  Enable : EnablePort
  To Workspace : ToWorkspace  VariableName=decoded  SampleTime=-1
      settings: Save2DSignal=2-D array (concatenate along first dimension)
  wires:
  In1/1 -> To Workspace/1

== system fec_ber_hw_V2/Encoder Ctrl/Rising Edge ==
  In1 : Inport
  Data Type Conversion1 : DataTypeConversion  OutDataTypeStr=boolean  SaturateOnIntegerOverflow=on  RndMeth=Zero
  Delay2 : Delay  DelayLength=1  InitialCondition=1  InputProcessing=Columns as channels (frame based)
  Logical Operator : Logic  Operator=NOT  Inputs=1
  Logical Operator1 : Logic
  Out1 : Outport
  wires:
  In1/1 -> Data Type Conversion1/1
  Data Type Conversion1/1 -> Logical Operator1/1, Delay2/1
  Logical Operator/1 -> Logical Operator1/2
  Delay2/1 -> Logical Operator/1
  Logical Operator1/1 -> Out1/1

== system fec_ber_hw_V2/QAM Mapping/Buffer ==
  s_axis_tvalid : Inport
  s_axis_tdata : Inport  Port=2
  AND1 : Logic  IconShape=distinctive  AllPortsSameDT=off  OutDataTypeStr=boolean
  Constant : Constant  Value=8190  OutDataTypeStr=fixdt(0,log2(8190),0)  SampleTime=-1
  Delay4 : Delay  DelayLength=1
  GreaterThan : RelationalOperator  Operator=<  OutDataTypeStr=boolean  RndMeth=Simplest
  HDL FIFO : hdlsllib/HDL RAMs/HDL FIFO  fifo_size=128  mode=Classic  ratio=1  push_msg=Warning  pop_msg=Warning  show_empty=on  show_full=on  show_num=on  LabelModeActiveChoice_Mode=Classic
      settings: SourceProductBaseCode=SL
  NOT : Logic  Operator=NOT  IconShape=distinctive  AllPortsSameDT=off  OutDataTypeStr=boolean
  NOT1 : Logic  Operator=NOT  IconShape=distinctive  AllPortsSameDT=off  OutDataTypeStr=boolean
  " m_axis_tvalid" : Outport
  " m_axis_tdata" : Outport  Port=2
  s_axis_tready : Outport  Port=3
  wires:
  HDL FIFO/1 -> " m_axis_tdata"/1
  Delay4/1 -> " m_axis_tvalid"/1
  GreaterThan/1 -> s_axis_tready/1
  HDL FIFO/2 -> NOT/1
  HDL FIFO/4 -> GreaterThan/1
  AND1/1 -> HDL FIFO/2
  HDL FIFO/3 -> NOT1/1
  Constant/1 -> GreaterThan/2
  NOT1/1 -> AND1/2
  s_axis_tvalid/1 -> AND1/1
  s_axis_tdata/1 -> HDL FIFO/1
  NOT/1 -> HDL FIFO/3, Delay4/1

== system fec_ber_hw_V2/QAM Mapping/QAM Mapping ==
  bits lane0 : Inport
  Enable : EnablePort
  N-Width QAM-16 Symbol Mapping Imag : Subsystem  mask{bits=64}
      mask prompts: bits "Width:"
      mask init:
      | top_block = gcb;
      | % set_param(top_block, 'LinkStatus', 'none');
      | 
      | block_names = find_system(top_block, 'LookUnderMasks','on', 'SearchDepth','1');
      | 
      | in_block = sprintf('%s/bits', top_block);
      | out_block = sprintf('%s/symbol', top_block);
      | qam_16_block = sprintf('%s/QAM-16 Symbol Mapping 0', top_block);
      | % enable_block = sprintf('%s/enable', n_qam_16);
      | 
      | keep_blocks = {top_block, in_block, out_block, qam_16_block};
      | 
      | for i = 1:length(block_names)
      |     if ~ismember(block_names{i}, keep_blocks)
      |         delete_block(block_names{i});
      |     end
      | end
      | delete_line(find_system(top_block,'LookUnderMasks', 'all','SearchDepth', '1', 'FindAll','on','type','line'));
      | 
      | % Add QAM-16 Mapping Blocks
      | pos = get_param(qam_16_block, 'position');
      | new_pos = pos;
      | set_param(qam_16_block, 'n', num2str(bits-4));
      | for bit = 4:4:bits-1
      |     new_block = sprintf('%s%d', qam_16_block(1:end-1), bit/4);
      |     add_block(qam_16_block, new_block);
      |     new_pos = pos + ([0 60 0 60] * (bit/4));
      |     set_param(new_block, 'position', new_pos);
      |     set_param(new_block, 'n', num2str(bits-4-bit));
      | end
      | 
      | % Add the Bit Concat
      | concat_block = sprintf('%s/concat', top_block);
      | add_block('hdlsllib/Logic and Bit Operations/Bit Concat', concat_block);
      | set_param(concat_block, 'numInputs', num2str(bits/4));
      | concat_position = new_pos + [175 0 175 0];
      | concat_position(2) = pos(2);
      | set_param(concat_block, 'position', concat_position);
      | 
      | % Reposition Input and Outputs
      | out_position = get_param(out_block, 'position');
      | height = out_position(4) - out_position(2);
      | width = out_position(3) - out_position(1);
      | middle_h = (concat_position(4) - concat_position(2))/2 + concat_position(2);
      | out_position = [concat_position(1) + 175, middle_h - height/2, concat_position(1) + 175 + width, middle_h + height/2];
      | set_param(out_block, 'position', out_position);
      | 
      | in_position = [concat_position(1) - 300, middle_h - height/2, concat_position(1) - 300 + width, middle_h + height/2];
      | set_param(in_block, 'position', in_position);
      | 
      | % enable_position = get_param(enable_block, 'position');
      | % set_param(enable_block, 'position', enable_position - [0 100 0 100]);
      | 
      | % Connect Ports
      | for bit = 1:4:bits
      |     add_line(top_block,'bits/1',sprintf('QAM-16 Symbol Mapping %d/1',(bit-1)/4));
      |     add_line(top_block,sprintf('QAM-16 Symbol Mapping %d/1',(bit-1)/4),sprintf('concat/%d', ceil(bit/4)));
      | %     add_line(top_block,sprintf('QAM-16 Symbol Mapping %d/2',(bit-1)/4),sprintf('concat/%d', ceil(bit/2)+1));
      | end
      | add_line(top_block,'concat/1','symbol/1');
  N-Width QAM-16 Symbol Mapping Real : Subsystem  mask{bits=64}
      mask prompts: bits "Width:"
      mask init: same as fec_ber_hw_V2/QAM Mapping/QAM Mapping/N-Width QAM-16 Symbol Mapping Imag
  Q symbols : Outport
  I symbols : Outport  Port=2
  wires:
  bits lane0/1 -> N-Width QAM-16 Symbol Mapping Imag/1(bits), N-Width QAM-16 Symbol Mapping Real/1(bits)
  N-Width QAM-16 Symbol Mapping Real/1(symbol) -> I symbols/1
  N-Width QAM-16 Symbol Mapping Imag/1(symbol) -> Q symbols/1
